simulink model "cruise_control"  (R2023b)
settings: Solver=VariableStepAuto  StartTime=0.0  StopTime=10  RelTol=1e-3
libraries: slpidlib x1, simulink x1
settings Model: Creator=foderking  LastModifiedBy=foderking

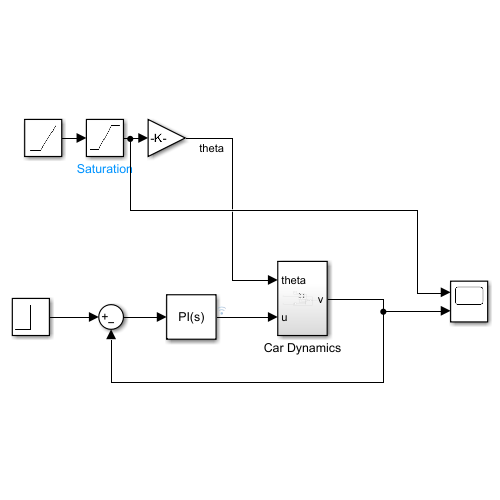
[thumbnail: Simulink's stored preview of the top-level diagram]
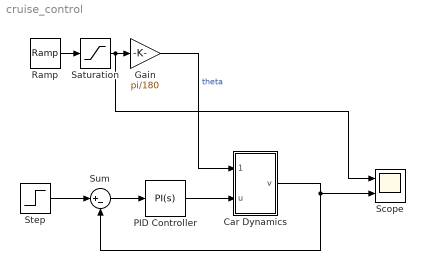
== system cruise_control ==
  Car Dynamics : Subsystem
  Gain : Gain  Gain=pi/180
  PID Controller : slpidlib/PID Controller  Controller=PI  Form=Parallel  TimeDomain=Continuous-time  UseExternalTs=off  SampleTime=-1  IntegratorMethod=Forward Euler  FilterMethod=Forward Euler  ControllerParametersSource=internal  P=0.5  I=0.1  UseKiTs=off  D=0  N=100  UseFilter=on  TunerSelectOption=Transfer Function Based (PID Tuner App)  InitialConditionSource=internal  InitialConditionForIntegrator=0  InitialConditionForFilter=0  DifferentiatorICPrevScaledInput=0  ExternalReset=none  TrackingMode=off  Kt=1  LimitOutput=off  SatLimitsSource=internal  UpperSaturationLimit=inf  LowerSaturationLimit=-inf  LinearizeAsGain=on  AntiWindupMode=none  Kb=1  LimitIntegrator=off  UpperIntegratorSaturationLimit=inf  LowerIntegratorSaturationLimit=-inf  POutMin=[]  POutMax=[]  IOutMin=[]  IOutMax=[]  DOutMin=[]  DOutMax=[]  NOutMin=[]  NOutMax=[]  SumOutMin=[]  SumOutMax=[]  SaturationOutMin=[]  SaturationOutMax=[]  PParamMin=[]  PParamMax=[]  IParamMin=[]  IParamMax=[]  DParamMin=[]  DParamMax=[]  NParamMin=[]  NParamMax=[]  KbParamMin=[]  KbParamMax=[]  KtParamMin=[]  KtParamMax=[]  KbOutMin=[]  KbOutMax=[]  KtOutMin=[]  KtOutMax=[]  IntegratorOutMin=[]  IntegratorOutMax=[]  FilterOutMin=[]  FilterOutMax=[]  SumI1OutMin=[]  SumI1OutMax=[]  SumI2OutMin=[]  SumI2OutMax=[]  SumI3OutMin=[]  SumI3OutMax=[]  SumI4OutMin=[]  SumI4OutMax=[]  SumDOutMin=[]  SumDOutMax=[]  DifferentiatorOutMin=[]  DifferentiatorOutMax=[]  FilterDiffOutCoefMin=[]  FilterDiffOutCoefMax=[]  ReciprocalOutMin=[]  ReciprocalOutMax=[]  SumDenOutMin=[]  SumDenOutMax=[]  SumNumOutMin=[]  SumNumOutMax=[]  DivideOutMin=[]  DivideOutMax=[]  UdiffTsProdOutMin=[]  UdiffTsProdOutMax=[]  NTsProdOutMin=[]  NTsProdOutMax=[]  UintegralTsProdOutMin=[]  UintegralTsProdOutMax=[]  UngainTsProdOutMin=[]  UngainTsProdOutMax=[]  ClampingZeroOutDataTypeStr=Inherit: Inherit via back propagation  ClampingZeroOutMin=[]  ClampingZeroOutMax=[]  FilterDenConstantOutDataTypeStr=Inherit: Inherit via back propagation  FilterDenConstantOutMin=[]  FilterDenConstantOutMax=[]  PCopyOutDataTypeStr=Inherit: Inherit via back propagation  PCopyOutMin=[]  PCopyOutMax=[]  NCopyOutDataTypeStr=Inherit: Inherit via back propagation  NCopyOutMin=[]  NCopyOutMax=[]  IntegratorContinuousStateAttributes=''  IntegratorStateMustResolveToSignalObject=off  IntegratorRTWStateStorageClass=Auto  FilterContinuousStateAttributes=''  FilterStateMustResolveToSignalObject=off  FilterRTWStateStorageClass=Auto  ParallelPVariant=InternalParameters  IdealPVariant=Disabled  IVariant=InternalParameters  DVariant=Disabled  IntegratorVariant=Continuous  SatVariant=Disabled  AWVariant=Passthrough  PCopyVariant=Disabled  TRVariant=Disabled  FdbkBlocksVariant=Forward  IdealPFdbkVariant=Disabled  SatFdbkVariant=Disabled  DerivativeFilterVariant=Disabled  NVariant=Disabled  NCopyVariant=Disabled_SignalSpec  FilterICVariant=Disabled  IntegratorICVariant=InternalICs  ExternalResetVariant=Disabled  TRSumVariant=Passthrough  SumFdbkVariant=Disabled  SumVariant=Sum_PI  TsampFilterVariant=InternalTs  TsampNgainVariant=Passthrough  TsampIntegralVariant=Disabled_SignalSpec  ExternalSaturationOutDataTypeStr=Inherit: Same as second input
  Ramp : simulink/Sources/Ramp  slope=0  start=5  InitialOutput=0
  Saturation : Saturate  UpperLimit=4
  Scope : Scope  NumInputPorts=2
  Step : Step  Time=0  After=20  SampleTime=0
  Sum : Sum  Inputs=|+-
  wires:
  Car Dynamics/1(v) -> Sum/2, Scope/2
  Ramp/1 -> Saturation/1
  Saturation/1 -> Scope/1, Gain/1
  Gain/1 -> Car Dynamics/1(theta)  "theta"
  PID Controller/1 -> Car Dynamics/2(u)
  Step/1 -> Sum/1
  Sum/1 -> PID Controller/1

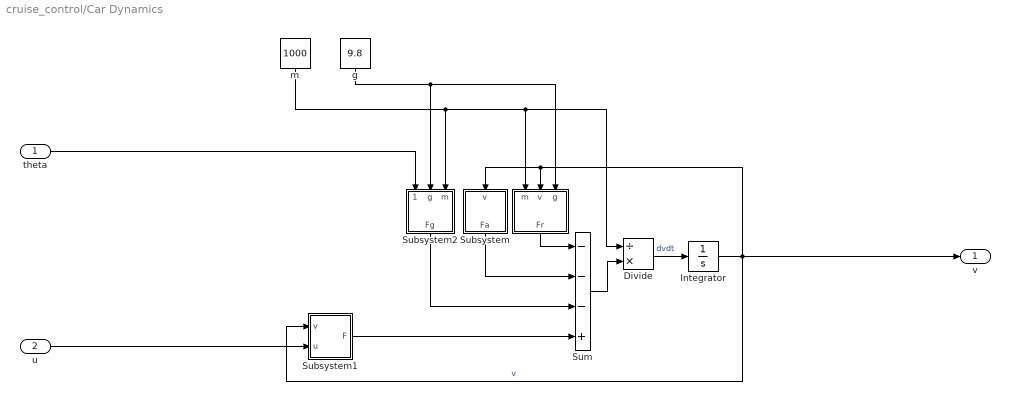
== system cruise_control/Car Dynamics ==
  theta : Inport
  u : Inport  Port=2
  " " : Subsystem
  Divide : Product  Inputs=/*
  Integrator : Integrator
  Subsystem : Subsystem
  Subsystem1 : Subsystem
  Subsystem2 : Subsystem
  Sum : Sum  Inputs=---+
  g : Constant  Value=9.8
  m : Constant  Value=1000
  v : Outport
  wires:
  m/1 -> Divide/1, " "/1(m), Subsystem2/3(m)
  Sum/1 -> Divide/2
  Divide/1 -> Integrator/1  "dvdt"
  " "/1(Fr) -> Sum/1
  Integrator/1 -> v/1, Subsystem/1(v), " "/2(v), Subsystem1/1(v)  "v"
  Subsystem/1(Fa) -> Sum/2
  Subsystem1/1(F) -> Sum/4
  u/1 -> Subsystem1/2(u)
  g/1 -> " "/3(g), Subsystem2/2(g)
  Subsystem2/1(Fg) -> Sum/3
  theta/1 -> Subsystem2/1(theta)

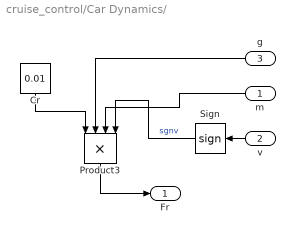
== system cruise_control/Car Dynamics/  ==
  m : Inport
  v : Inport  Port=2
  g : Inport  Port=3
  Cr : Constant  Value=0.01
  Product3 : Product  Inputs=4
  Sign : Signum
  Fr : Outport
  wires:
  Cr/1 -> Product3/1
  g/1 -> Product3/2
  Product3/1 -> Fr/1
  v/1 -> Sign/1
  m/1 -> Product3/3
  Sign/1 -> Product3/4  "sgnv"

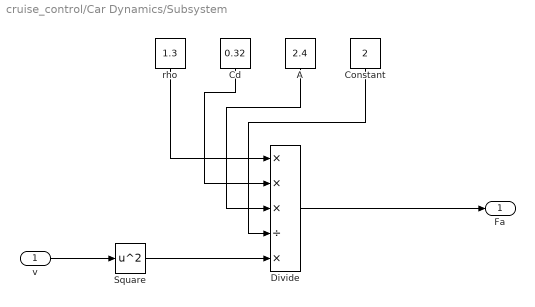
== system cruise_control/Car Dynamics/Subsystem ==
  v : Inport
  A : Constant  Value=2.4
  Cd : Constant  Value=0.32
  Constant : Constant  Value=2
  Divide : Product  Inputs=***/*
  Square : Math  Operator=square
  rho : Constant  Value=1.3
  Fa : Outport
  wires:
  v/1 -> Square/1
  rho/1 -> Divide/1
  A/1 -> Divide/3
  Cd/1 -> Divide/2
  Constant/1 -> Divide/4
  Square/1 -> Divide/5
  Divide/1 -> Fa/1

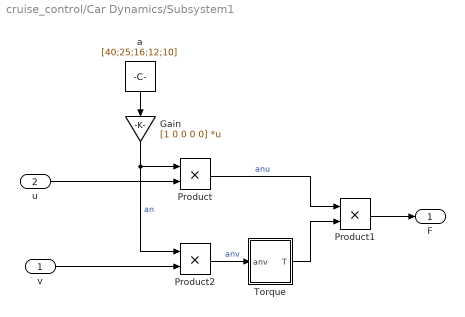
== system cruise_control/Car Dynamics/Subsystem1 ==
  v : Inport
  u : Inport  Port=2
  Gain : Gain  Gain=[1 0 0 0 0]  Multiplication=Matrix(K*u)
  Product : Product
  Product1 : Product
  Product2 : Product
  Torque : Subsystem
  a : Constant  Value=[40;25;16;12;10]
  F : Outport
  wires:
  a/1 -> Gain/1
  Product2/1 -> Torque/1(anv)  "anv"
  Torque/1(T) -> Product1/2
  Product/1 -> Product1/1  "anu"
  Gain/1 -> Product2/1, Product/1  "an"
  u/1 -> Product/2
  Product1/1 -> F/1
  v/1 -> Product2/2

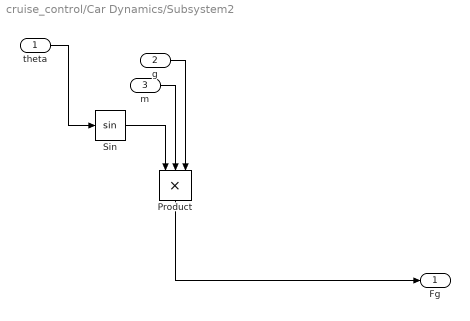
== system cruise_control/Car Dynamics/Subsystem2 ==
  theta : Inport
  g : Inport  Port=2
  m : Inport  Port=3
  Product : Product  Inputs=3
  Sin : Trigonometry
  Fg : Outport
  wires:
  Sin/1 -> Product/1
  Product/1 -> Fg/1
  theta/1 -> Sin/1
  m/1 -> Product/2
  g/1 -> Product/3

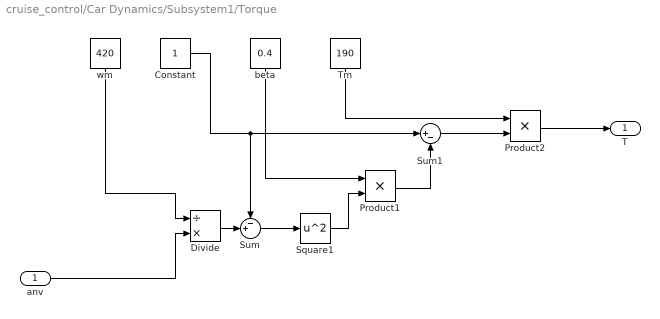
== system cruise_control/Car Dynamics/Subsystem1/Torque ==
  anv : Inport
  Constant : Constant
  Divide : Product  Inputs=/*
  Product1 : Product
  Product2 : Product
  Square1 : Math  Operator=square
  Sum : Sum  Inputs=-+|
  Sum1 : Sum  Inputs=|+-
  Tm : Constant  Value=190
  beta : Constant  Value=0.4
  wm : Constant  Value=420
  T : Outport
  wires:
  beta/1 -> Product1/1
  Tm/1 -> Product2/1
  wm/1 -> Divide/1
  anv/1 -> Divide/2
  Divide/1 -> Sum/2
  Constant/1 -> Sum/1, Sum1/1
  Sum/1 -> Square1/1
  Square1/1 -> Product1/2
  Product1/1 -> Sum1/2
  Sum1/1 -> Product2/2
  Product2/1 -> T/1
